simulink model "untitledservo2"  (R2016a)
settings: Solver=VariableStepAuto  StartTime=0.0  StopTime=10.0  RelTol=1e-3
libraries: arduinolib x6
settings Model: Creator=mezia  LastModifiedBy=mezia

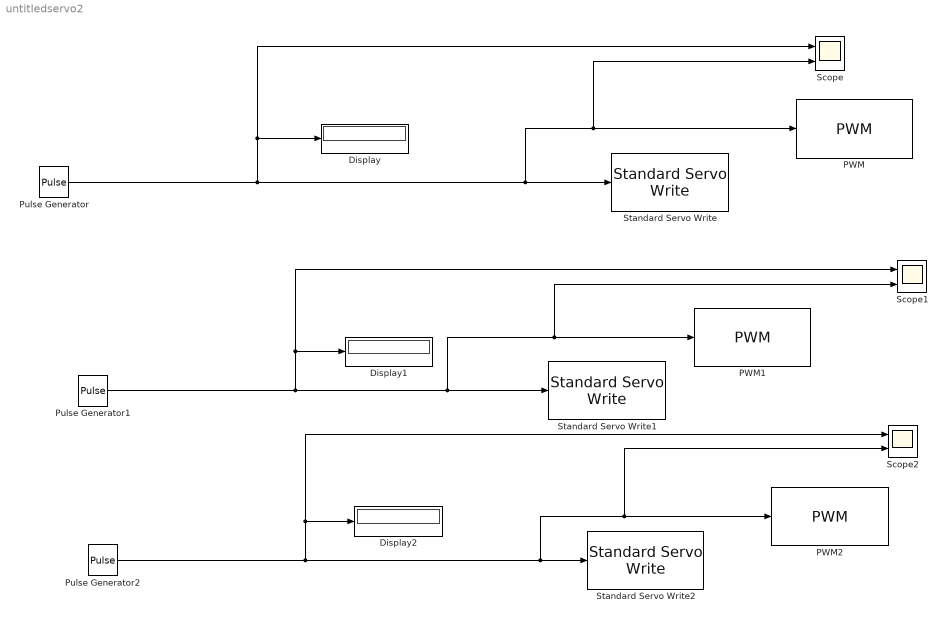
== system untitledservo2 ==
  Display : Display
  Display1 : Display
  Display2 : Display
  PWM : arduinolib/PWM  pinNumber=9  blockPlatform=arduino
  PWM1 : arduinolib/PWM  pinNumber=5  blockPlatform=arduino
  PWM2 : arduinolib/PWM  pinNumber=6  blockPlatform=arduino
  Pulse Generator : DiscretePulseGenerator  Amplitude=180  Period=20  PulseWidth=10  SampleTime=0.1
  Pulse Generator1 : DiscretePulseGenerator  Amplitude=180  Period=20  PulseWidth=10  SampleTime=0.1
  Pulse Generator2 : DiscretePulseGenerator  Amplitude=180  Period=20  PulseWidth=10  SampleTime=0.1
  Scope : Scope  NumInputPorts=2
  Scope1 : Scope  NumInputPorts=2
  Scope2 : Scope  NumInputPorts=2
  Standard Servo Write : arduinolib/Standard Servo Write  pinNumber=9  blockPlatform=arduino
  Standard Servo Write1 : arduinolib/Standard Servo Write  pinNumber=5  blockPlatform=arduino
  Standard Servo Write2 : arduinolib/Standard Servo Write  pinNumber=6  blockPlatform=arduino
  wires:
  Pulse Generator/1 -> Scope/2, PWM/1, Standard Servo Write/1, Scope/1, Display/1
  Pulse Generator1/1 -> Scope1/2, PWM1/1, Standard Servo Write1/1, Scope1/1, Display1/1
  Pulse Generator2/1 -> Scope2/2, PWM2/1, Standard Servo Write2/1, Scope2/1, Display2/1
